simulink model "Ackerman_build"  (R2020a)
settings: Solver=VariableStepAuto  StartTime=0.0  StopTime=10.0  RelTol=1e-3
model workspace (MAT data in the model file):
  theta = Simulink.Parameter
  theta.DataType = 'double'
  theta.Dimensions = [0 0]
settings Model: OrderedModelArguments=off  Creator=João Fernando Rangel  LastModifiedBy=João Fernando Rangel

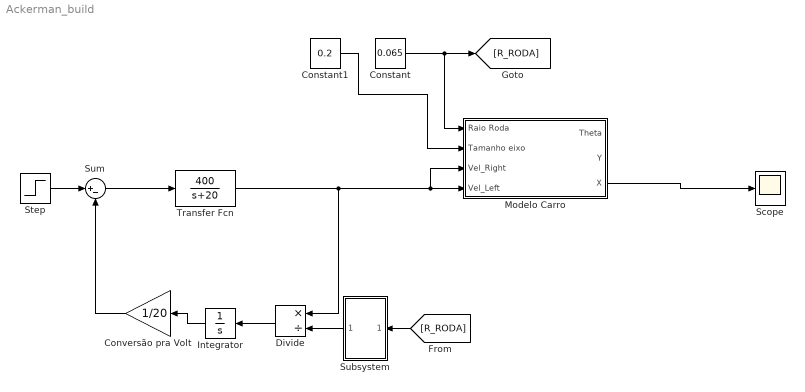
== system Ackerman_build ==
  Constant : Constant  Value=0.065
  Constant1 : Constant  Value=0.2
  Conversão pra Volt : Gain  Gain=1/20
  Divide : Product  Inputs=*/
  Integrator : Integrator
  Modelo Carro : Subsystem
  Scope : Scope
  Step : Step  Time=0  After=20  SampleTime=0
  Subsystem : Subsystem
  Sum : Sum  Inputs=|+-
  Transfer Fcn : TransferFcn  Numerator=[400]  Denominator=[1 20]
  wires:
  Constant/1 -> [R_RODA], Modelo Carro/1(Raio Roda)
  Constant1/1 -> Modelo Carro/2(Tamanho eixo)
  Transfer Fcn/1 -> Divide/1, Modelo Carro/3(Vel_Right), Modelo Carro/4(Vel_Left)
  Sum/1 -> Transfer Fcn/1
  Step/1 -> Sum/1
  Conversão pra Volt/1 -> Sum/2
  Divide/1 -> Integrator/1
  Integrator/1 -> Conversão pra Volt/1
  [R_RODA] -> Subsystem/1(In1)
  Subsystem/1(Out1) -> Divide/2
  Modelo Carro/3(X) -> Scope/1

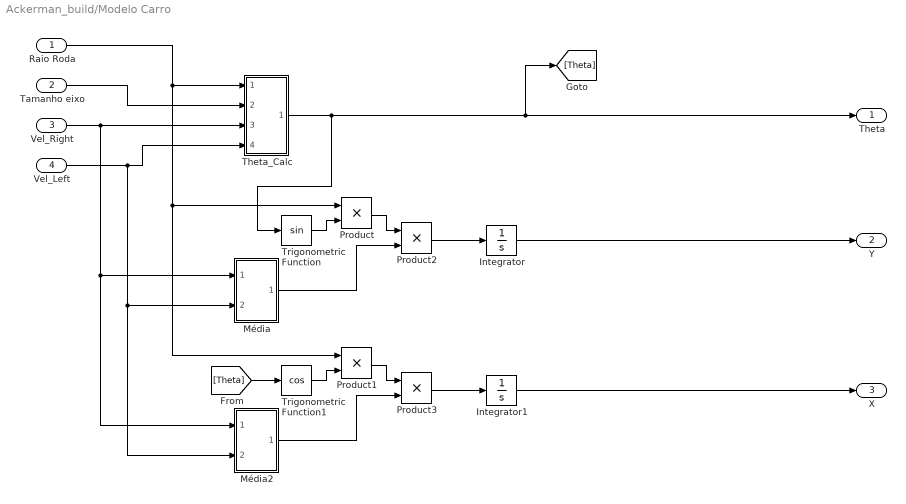
== system Ackerman_build/Modelo Carro ==
  Raio Roda : Inport
  Tamanho eixo : Inport  Port=2
  Vel_Right : Inport  Port=3
  Vel_Left : Inport  Port=4
  Integrator : Integrator
  Integrator1 : Integrator
  Média : Subsystem
  Média2 : Subsystem
  Product{,1..3} (4 alike) : Product
  Theta_Calc : Subsystem
  Trigonometric Function : Trigonometry
  Trigonometric Function1 : Trigonometry  Operator=cos
  Theta : Outport
  Y : Outport  Port=2
  X : Outport  Port=3
  wires:
  Vel_Right/1 -> Média2/1(Vel_Right), Média/1(In1), Theta_Calc/3(In3)
  Média/1(Out1) -> Product2/2
  Vel_Left/1 -> Média2/2(Vel_Left), Média/2(In2), Theta_Calc/4(In4)
  Raio Roda/1 -> Product1/1, Product/1, Theta_Calc/1(In1)
  Trigonometric Function/1 -> Product/2
  [Theta] -> Trigonometric Function1/1
  Tamanho eixo/1 -> Theta_Calc/2(In2)
  Trigonometric Function1/1 -> Product1/2
  Média2/1(Out1) -> Product3/2
  Theta_Calc/1(Out1) -> Trigonometric Function/1, Theta/1, [Theta]
  Integrator1/1 -> X/1
  Product2/1 -> Integrator/1
  Product/1 -> Product2/1
  Integrator/1 -> Y/1
  Product3/1 -> Integrator1/1
  Product1/1 -> Product3/1

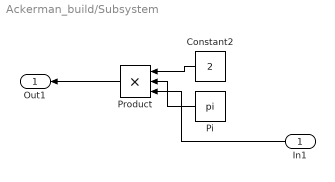
== system Ackerman_build/Subsystem ==
  In1 : Inport
  Constant2 : Constant  Value=2
  Pi : Constant  Value=pi  OutDataTypeStr=Inherit: Inherit via back propagation
  Product : Product  Inputs=3
  Out1 : Outport
  wires:
  Constant2/1 -> Product/1
  Pi/1 -> Product/2
  Product/1 -> Out1/1
  In1/1 -> Product/3

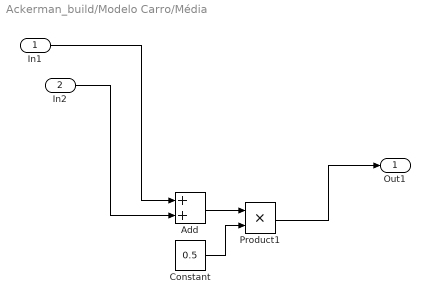
== system Ackerman_build/Modelo Carro/Média ==
  In1 : Inport
  In2 : Inport  Port=2
  Add : Sum
  Constant : Constant  Value=0.5
  Product1 : Product
  Out1 : Outport
  wires:
  Constant/1 -> Product1/2
  Add/1 -> Product1/1
  In2/1 -> Add/2
  Product1/1 -> Out1/1
  In1/1 -> Add/1

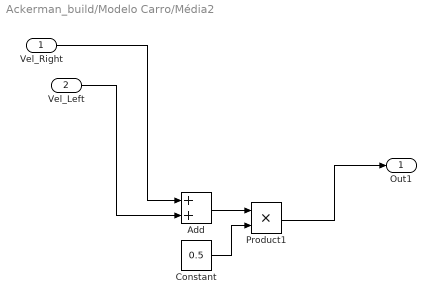
== system Ackerman_build/Modelo Carro/Média2 ==
  Vel_Right : Inport
  Vel_Left : Inport  Port=2
  Add : Sum
  Constant : Constant  Value=0.5
  Product1 : Product
  Out1 : Outport
  wires:
  Constant/1 -> Product1/2
  Add/1 -> Product1/1
  Vel_Left/1 -> Add/2
  Product1/1 -> Out1/1
  Vel_Right/1 -> Add/1

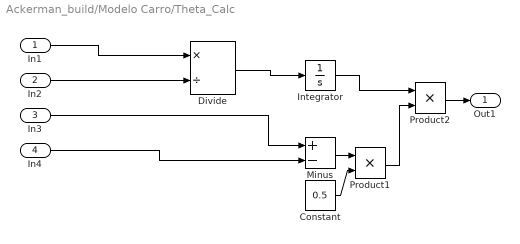
== system Ackerman_build/Modelo Carro/Theta_Calc ==
  In1 : Inport
  In2 : Inport  Port=2
  In3 : Inport  Port=3
  In4 : Inport  Port=4
  Constant : Constant  Value=0.5
  Divide : Product  Inputs=*/
  Integrator : Integrator
  Minus : Sum  Inputs=+-
  Product1 : Product
  Product2 : Product
  Out1 : Outport
  wires:
  In3/1 -> Minus/1
  Product1/1 -> Product2/2
  Minus/1 -> Product1/1
  In4/1 -> Minus/2
  In2/1 -> Divide/2
  Product2/1 -> Out1/1
  Constant/1 -> Product1/2
  In1/1 -> Divide/1
  Divide/1 -> Integrator/1
  Integrator/1 -> Product2/1
